simulink model "Visualization"  (R2015a)
settings: Solver=FixedStepDiscrete  SolverMode=SingleTasking  StartTime=0.0  StopTime=inf  FixedStep=0.001  MaxStep=0.004  RelTol=1e-3
undefined symbols (not defined in the file or in its folder): gcbh, vrmfunc
libraries: dspsigops x2
settings Model: CovSFcnEnable=off  Creator=ADAM  LastModifiedBy=denise
settings SolverCC: ExtrapolationOrder=1
settings DataIOCC: LimitDataPoints=off  MaxDataPoints=1  SaveFormat=Structure  SignalLoggingSaveFormat=ModelDataLogs  SaveOutput=off  SignalLogging=off  DSMLogging=off  SaveTime=off  OutputSaveName=model_out  SignalLoggingName=model_out
settings OptimizationCC: ExpressionDepthLimit=2147483647  SimCompilerOptimization=on
settings DebuggingCC: UnderspecifiedInitializationDetection=Classic  MergeDetectMultiDrivingBlocksExec=none  SolverPrmCheckMsg=warning  InheritedTsInSrcMsg=none  MultiTaskDSMMsg=warning  MultiTaskCondExecSysMsg=none  UnconnectedInputMsg=none  UnconnectedOutputMsg=none  UnconnectedLineMsg=none  StateNameClashWarn=warning
settings HardwareCC: ProdIntDivRoundTo=Zero  ProdEndianess=LittleEndian  ProdHWDeviceType=Generic->32-bit x86 compatible
settings CodeAppCC: MaxIdLength=95

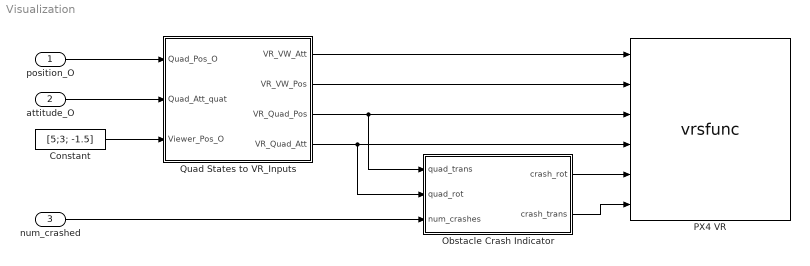
== system Visualization ==
  position_O : Inport  OutDataTypeStr=double  PortDimensions=3  SampleTime=0
  attitude_O : Inport  Port=2  OutDataTypeStr=double  PortDimensions=4  SampleTime=0
  num_crashed : Inport  Port=3  OutDataTypeStr=double  PortDimensions=1  SampleTime=0
  Constant : Constant  Value=[5;3; -1.5]  VectorParams1D=off
  Obstacle Crash Indicator : Subsystem
  PX4 VR : S-Function  InstantiateOnLoad=on  LoadFcn=vrmfunc('FnLoad', gcbh);  InitFcn=vrmfunc('FnInit', gcbh);  StartFcn=vrmfunc('FnSimStatus', gcbh, 'running')  StopFcn=vrmfunc('FnStop', gcbh)  FunctionName=vrsfunc  Parameters=SampleTime, VideoDimensions, 0  mask(Virtual Reality Sink){SampleTime=0.04, ViewEnable=on, RemoteChange=off, RemoteView=off, FieldsWritten=VW_Standing.orientation.4.1.1.double#VW_Standing.position.3.1.1.double#Quad_group.translation.3.1.1.double#Quad.rotation.4.1.1.double#crash.rotation.4.1.1.double#crash.translation.3.1.1.double, WorldFileName=px4.wrl, WorldDescription=TUW Field, AutoView=off, VideoDimensions=[], AllowVariableSize=off, FigureProperties=}
      mask prompts: SampleTime "Sample Time"; ViewEnable "View"; RemoteChange "Remote Change"; RemoteView "Remote View"; FieldsWritten "Fields Written"; WorldFileName "World File Name"; WorldDescription "World Description"; VideoDimensions "Video Dimensions"; AllowVariableSize "Allow Variable Size"; FigureProperties "Figure Properties"
      mask help: Controls the selected fields of a virtual world according to given inputs.
      mask init:
      | set_param(gcbh, 'MaskDisplay', vrmfunc('FnIcon'));
      settings: CopyFcn=vrmfunc('FnCopy', gcbh);  DeleteFcn=vrmfunc('FnDelete', gcbh);  PreSaveFcn=vrmfunc('FnPreSave', gcbh);  PauseFcn=vrmfunc('FnSimStatus', gcbh, 'paused');  ContinueFcn=vrmfunc('FnSimStatus', gcbh, 'running');  DestroyFcn=vrmfunc('FnDestroy', gcbh);  OpenFcn=vrmfunc('FnOpen', gcbh);  CloseFcn=vrmfunc('FnClose', gcbh);
      mask Help: helpview(vrmfunc('FnHelpTopic'), 'vr_vrsink');
      mask Display:
      | image(imread('vrblockicon.png'));
      | port_label('input', 1, 'VW_Standing.orientation');
      | port_label('input', 2, 'VW_Standing.position');
      | port_label('input', 3, 'Quad_group.translation');
      | port_label('input', 4, 'Quad.rotation');
      | port_label('input', 5, 'crash.rotation');
      | port_label('input', 6, 'crash.translation');
  Quad States to VR_Inputs : Subsystem
  wires:
  Constant/1 -> Quad States to VR_Inputs/3(Viewer_Pos_O)
  position_O/1 -> Quad States to VR_Inputs/1(Quad_Pos_O)
  attitude_O/1 -> Quad States to VR_Inputs/2(Quad_Att_quat)
  Quad States to VR_Inputs/1(VR_VW_Att) -> PX4 VR/1
  Quad States to VR_Inputs/2(VR_VW_Pos) -> PX4 VR/2
  Quad States to VR_Inputs/3(VR_Quad_Pos) -> Obstacle Crash Indicator/1(quad_trans), PX4 VR/3
  Quad States to VR_Inputs/4(VR_Quad_Att) -> Obstacle Crash Indicator/2(quad_rot), PX4 VR/4
  num_crashed/1 -> Obstacle Crash Indicator/3(num_crashes)
  Obstacle Crash Indicator/2(crash_trans) -> PX4 VR/6
  Obstacle Crash Indicator/1(crash_rot) -> PX4 VR/5

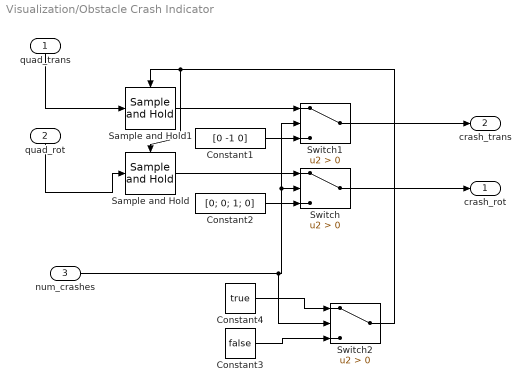
== system Visualization/Obstacle Crash Indicator ==
  quad_trans : Inport
  quad_rot : Inport  Port=2
  num_crashes : Inport  Port=3
  Constant1 : Constant  Value=[0 -1 0]  VectorParams1D=off
  Constant2 : Constant  Value=[0; 0; 1; 0]  VectorParams1D=off
  Constant3 : Constant  Value=false
  Constant4 : Constant  Value=true
  Sample and Hold : dspsigops/Sample and Hold  trig=Rising edge  initCond=0  latchinput=off
  Sample and Hold1 : dspsigops/Sample and Hold  trig=Rising edge  initCond=0  latchinput=off
  Switch : Switch  Criteria=u2 > Threshold
  Switch1 : Switch  Criteria=u2 > Threshold
  Switch2 : Switch  Criteria=u2 > Threshold
  crash_rot : Outport
  crash_trans : Outport  Port=2
  wires:
  Sample and Hold/1 -> Switch/1
  quad_trans/1 -> Sample and Hold1/1
  Constant4/1 -> Switch2/1
  Sample and Hold1/1 -> Switch1/1
  Constant3/1 -> Switch2/3
  Constant1/1 -> Switch1/3
  Switch1/1 -> crash_trans/1
  num_crashes/1 -> Switch2/2, Switch1/2, Switch/2
  Constant2/1 -> Switch/3
  Switch/1 -> crash_rot/1
  Switch2/1 -> Sample and Hold1/Trigger, Sample and Hold/Trigger
  quad_rot/1 -> Sample and Hold/1

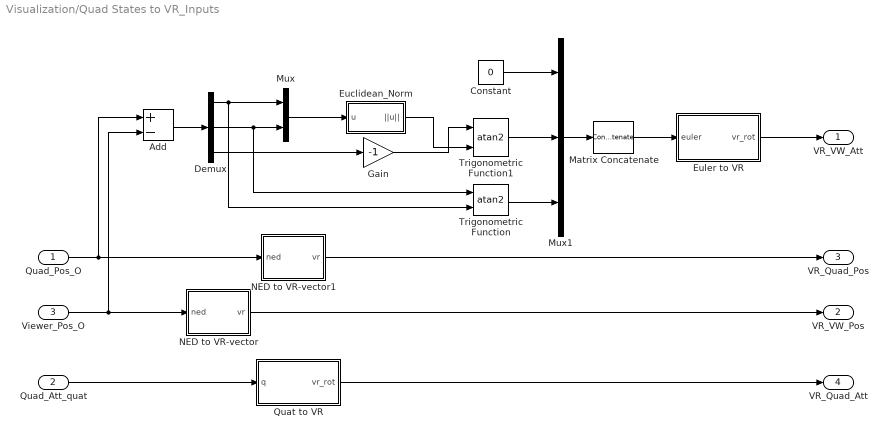
== system Visualization/Quad States to VR_Inputs ==
  Quad_Pos_O : Inport
  Quad_Att_quat : Inport  Port=2
  Viewer_Pos_O : Inport  Port=3
  Add : Sum  Inputs=+-
  Constant : Constant  Value=0
  Demux : Demux  Outputs=3
  Euclidean_Norm : Subsystem
      mask help: Euclidean Norm
      mask Help: Euclidean Norm
      mask Display: disp('||.||')
  Euler to VR : Subsystem  mask(Euler oritentation to VR-rotation){}
      mask help:
      | Converts a vector of euler angles to a VR-rotation.
      |
      | 1st rotation: psi   (=eul(1)) around z
      | 2nd rotation: theta (=eul(2)) around y
      | 3rd rotation: phi   (=eul(3)) around x
  Gain : Gain  Gain=-1
  Matrix Concatenate : Concatenate  NumInputs=1  Mode=Multidimensional array
  Mux : Mux  Inputs=2
  Mux1 : Mux  Inputs=3
  NED to VR-vector : Subsystem  mask(Converts NED to VR-vector){}
      mask help: [north east down] => [east up south]
  NED to VR-vector1 : Subsystem  mask(Converts NED to VR-vector){}
      mask help: [north east down] => [east up south]
  Quat to VR : Subsystem  mask(Quaternion to VR-rotation){}
      mask help: Converts a normalized quaternion to a VR-rotation.
  Trigonometric Function : Trigonometry  Operator=atan2
  Trigonometric Function1 : Trigonometry  Operator=atan2
  VR_VW_Att : Outport
  VR_VW_Pos : Outport  Port=2
  VR_Quad_Pos : Outport  Port=3
  VR_Quad_Att : Outport  Port=4
  wires:
  Trigonometric Function1/1 -> Mux1/2
  Trigonometric Function/1 -> Mux1/3
  Constant/1 -> Mux1/1
  Matrix Concatenate/1 -> Euler to VR/1(euler)
  Gain/1 -> Trigonometric Function1/1
  Demux/3 -> Gain/1
  Demux/1 -> Mux/1, Trigonometric Function/2
  Demux/2 -> Mux/2, Trigonometric Function/1
  NED to VR-vector/1(vr) -> VR_VW_Pos/1
  NED to VR-vector1/1(vr) -> VR_Quad_Pos/1
  Mux1/1 -> Matrix Concatenate/1
  Euler to VR/1(vr_rot) -> VR_VW_Att/1
  Mux/1 -> Euclidean_Norm/1(u)
  Euclidean_Norm/1(||u||) -> Trigonometric Function1/2
  Add/1 -> Demux/1
  Quad_Pos_O/1 -> Add/1, NED to VR-vector1/1(ned)
  Quat to VR/1(vr_rot) -> VR_Quad_Att/1
  Quad_Att_quat/1 -> Quat to VR/1(q)
  Viewer_Pos_O/1 -> Add/2, NED to VR-vector/1(ned)

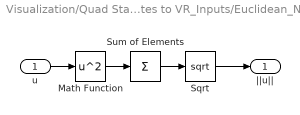
== system Visualization/Quad States to VR_Inputs/Euclidean_Norm ==
  u : Inport
  Math Function : Math  Operator=square  SaturateOnIntegerOverflow=on
  Sqrt : Sqrt  SaturateOnIntegerOverflow=on
  Sum of Elements : Sum  Inputs=+
  ||u|| : Outport
  wires:
  Sqrt/1 -> ||u||/1
  Sum of Elements/1 -> Sqrt/1
  Math Function/1 -> Sum of Elements/1
  u/1 -> Math Function/1

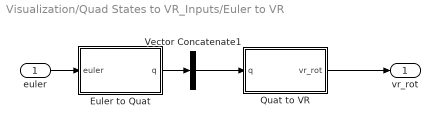
== system Visualization/Quad States to VR_Inputs/Euler to VR ==
  euler : Inport
  Euler to Quat : Subsystem  mask(Euler angles to Quaternion){}
      mask help:
      | vector [phi; theta; psi] means:
      | 1. rotation: psi   (=eul(3)) around z axis
      | 2. rotation: theta (=eul(2)) around y axis
      | 3. rotation: phi   (=eul(1)) around x axis
      |
      | Regrettably implemented in Simulink
  Quat to VR : Subsystem  mask(Quaternion to VR-rotation){}
      mask help: Converts a normalized quaternion to a VR-rotation.
  Vector Concatenate1 : Concatenate  NumInputs=1  Mode=Multidimensional array
  vr_rot : Outport
  wires:
  Quat to VR/1(vr_rot) -> vr_rot/1
  Euler to Quat/1(q) -> Vector Concatenate1/1
  euler/1 -> Euler to Quat/1(euler)
  Vector Concatenate1/1 -> Quat to VR/1(q)

== system Visualization/Quad States to VR_Inputs/NED to VR-vector ==
  ned : Inport
  Gain K*u : Gain  Gain=[0 1 0; 0 0 -1; -1 0 0]  Multiplication=Matrix(K*u)
  vr : Outport
  wires:
  Gain K*u/1 -> vr/1
  ned/1 -> Gain K*u/1

== system Visualization/Quad States to VR_Inputs/NED to VR-vector1 ==
  ned : Inport
  Gain K*u : Gain  Gain=[0 1 0; 0 0 -1; -1 0 0]  Multiplication=Matrix(K*u)
  vr : Outport
  wires:
  Gain K*u/1 -> vr/1
  ned/1 -> Gain K*u/1

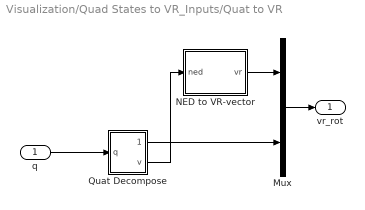
== system Visualization/Quad States to VR_Inputs/Quat to VR ==
  q : Inport
  Mux : Mux  Inputs=2
  NED to VR-vector : Subsystem  mask(Converts NED to VR-vector){}
      mask help: [north east down] => [east up south]
  Quat Decompose : Subsystem  mask(Quaternion Decomposition){}
      mask help:
      | Decomposes a normalized Quaternion into
      | the rotation-vector v and the rotation-angle phi.
  vr_rot : Outport
  wires:
  q/1 -> Quat Decompose/1(q)
  Quat Decompose/2(v) -> NED to VR-vector/1(ned)
  NED to VR-vector/1(vr) -> Mux/1
  Quat Decompose/1(phi) -> Mux/2
  Mux/1 -> vr_rot/1

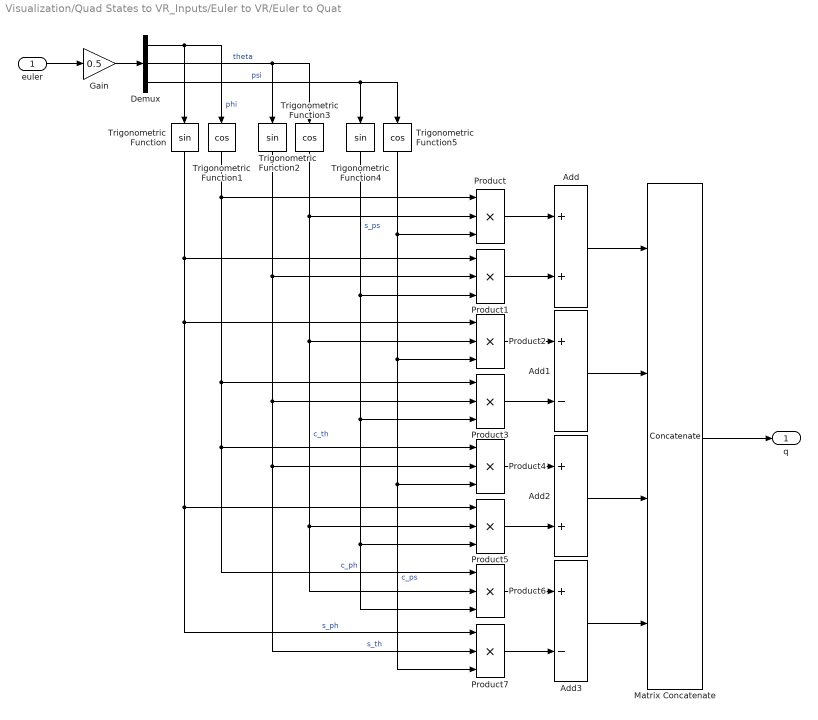
== system Visualization/Quad States to VR_Inputs/Euler to VR/Euler to Quat ==
  euler : Inport
  Add : Sum
  Add1 : Sum  Inputs=+-
  Add2 : Sum
  Add3 : Sum  Inputs=+-
  Demux : Demux  Outputs=3
  Gain : Gain  Gain=0.5
  Matrix Concatenate : Concatenate  NumInputs=4  ConcatenateDimension=2
  Product{,1..7} (8 alike) : Product  Inputs=3  RndMeth=Zero
  Trigonometric Function : Trigonometry
  Trigonometric Function1 : Trigonometry  Operator=cos
  Trigonometric Function2 : Trigonometry
  Trigonometric Function3 : Trigonometry  Operator=cos
  Trigonometric Function4 : Trigonometry
  Trigonometric Function5 : Trigonometry  Operator=cos
  q : Outport
  wires:
  Trigonometric Function1/1 -> Product/1, Product3/1, Product4/1, Product6/1  "c_ph"
  Trigonometric Function3/1 -> Product/2, Product2/2, Product5/2, Product6/2  "c_th"
  Trigonometric Function4/1 -> Product1/3, Product3/3, Product5/3, Product6/3  "s_ps"
  Trigonometric Function/1 -> Product1/1, Product2/1, Product5/1, Product7/1  "s_ph"
  Trigonometric Function2/1 -> Product1/2, Product3/2, Product4/2, Product7/2  "s_th"
  Trigonometric Function5/1 -> Product/3, Product2/3, Product4/3, Product7/3  "c_ps"
  Matrix Concatenate/1 -> q/1
  Add3/1 -> Matrix Concatenate/4
  Add2/1 -> Matrix Concatenate/3
  Add1/1 -> Matrix Concatenate/2
  Add/1 -> Matrix Concatenate/1
  Product7/1 -> Add3/2
  Product6/1 -> Add3/1
  Product5/1 -> Add2/2
  Product4/1 -> Add2/1
  Product3/1 -> Add1/2
  Product2/1 -> Add1/1
  Product1/1 -> Add/2
  Product/1 -> Add/1
  Demux/1 -> Trigonometric Function1/1, Trigonometric Function/1  "phi"
  Demux/2 -> Trigonometric Function3/1, Trigonometric Function2/1  "theta"
  Demux/3 -> Trigonometric Function5/1, Trigonometric Function4/1  "psi"
  Gain/1 -> Demux/1
  euler/1 -> Gain/1

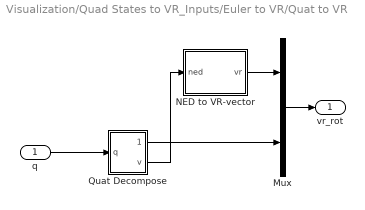
== system Visualization/Quad States to VR_Inputs/Euler to VR/Quat to VR ==
  q : Inport
  Mux : Mux  Inputs=2
  NED to VR-vector : Subsystem  mask(Converts NED to VR-vector){}
      mask help: [north east down] => [east up south]
  Quat Decompose : Subsystem  mask(Quaternion Decomposition){}
      mask help:
      | Decomposes a normalized Quaternion into
      | the rotation-vector v and the rotation-angle phi.
  vr_rot : Outport
  wires:
  q/1 -> Quat Decompose/1(q)
  Quat Decompose/2(v) -> NED to VR-vector/1(ned)
  NED to VR-vector/1(vr) -> Mux/1
  Quat Decompose/1(phi) -> Mux/2
  Mux/1 -> vr_rot/1

== system Visualization/Quad States to VR_Inputs/Quat to VR/NED to VR-vector ==
  ned : Inport
  Gain K*u : Gain  Gain=[0 1 0; 0 0 -1; -1 0 0]  Multiplication=Matrix(K*u)
  vr : Outport
  wires:
  Gain K*u/1 -> vr/1
  ned/1 -> Gain K*u/1

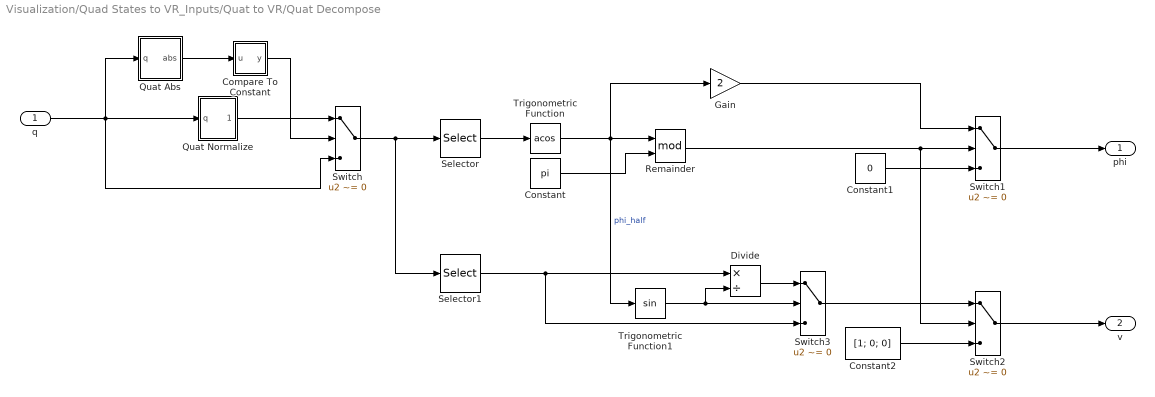
== system Visualization/Quad States to VR_Inputs/Quat to VR/Quat Decompose ==
  q : Inport
  Compare To Constant : Subsystem  mask(Compare To Constant){relop=~=, const=1, OutDataTypeStr=uint8, ZeroCross=off}
      mask prompts: relop "Simulink:masks:Operator_MP"; const "Simulink:masks:ConstantValue_MP"; OutDataTypeStr "Simulink:masks:OutputDataType_MP"; ZeroCross "Simulink:masks:EnableZerocrossingDetection_MP"
      mask help: Simulink:masks:CompareToConstant_MD
      mask init:
      | blkName = gcb;
      | 
      | if strcmp(get_param(gcbh,'OutDataTypeStr'),'boolean')
      | 	setValue = 'boolean';
      | else
      | 	setValue = 'fixdt(0, 8)';
      | end
      | 
      | set_param([blkName,'/Compare'],'relop',relop, ...
      | 	'OutDataTypeStr', setValue, 'ZeroCross', ZeroCross);
      | 
      | str = [relop,' C']; %default
      | 
      | const_str = get_param(blkName, 'const');
      | 
      | if isempty(strfind(const_str, ' ')) && isempty(strfind(const_str, ','))
      |     % scalar or single expression
      |     if isempty(str2num(const_str))
      |         %expression
      |         str = [relop, ' ', const_str];
      |     elseif length(const) == 1
      |         str = [relop,' ',num2str(double(const))];
      |     end
      | end
      mask TypeOptions relop: == | ~= | < | <= | >= | >
      mask TypeOptions OutDataTypeStr: Simulink:masks:uint8 | Simulink:masks:boolean
      mask Callback ZeroCross: sl('zeroCrossEnable', gcbh);
      mask Display: disp(str)
  Constant : Constant  Value=pi  OutDataTypeStr=Inherit: Inherit via back propagation
  Constant1 : Constant  Value=0  VectorParams1D=off
  Constant2 : Constant  Value=[1; 0; 0]  VectorParams1D=off
  Divide : Product  Inputs=*/
  Gain : Gain  Gain=2
  Quat Abs : Subsystem  mask(Absolute value){}
      mask help: sqrt(q(1)^2+q(2)^2+q(3)^2+q(4)^2)
      mask init:
      | pos = get_param(gcb, 'Position');
      | width = pos(3) - pos(1); height = pos(4) - pos(2);
      | fontsize = get_param(gcb, 'fontsize');
      | if fontsize==-1, scale=1; else scale=fontsize/10; end
      mask Display: text(width/2-scale*8, (height/2-scale), '||q||')
  Quat Normalize : Subsystem  mask(Quaternion Normalize){}
      mask help:
      | if abs(q) ~= 0
      |     q_norm = q/sqrt(q(1)^2+q(2)^2+q(3)^2+q(4)^2)
      | else
      |     q_norm = [1; 0; 0; 0]
      |
      | Regrettably implemented in Simulink
      mask init:
      | pos = get_param(gcb, 'Position');
      | width = pos(3) - pos(1); height = pos(4) - pos(2);
      | fontsize = get_param(gcb, 'fontsize');
      | if fontsize==-1, scale=1; else scale=fontsize/10; end
      mask Display:
      | text(width/2-scale*3, (height/2+scale*10), 'q')
      | text(width/2-scale*8, (height/2-scale*6), '||q||')
      | plot([width/2-scale*10 width/2+scale*10], height/2*[1 1])
  Remainder : Math  Operator=mod  SaturateOnIntegerOverflow=on
  Selector : Selector  InputPortWidth=4  Indices=[1]
  Selector1 : Selector  InputPortWidth=4  Indices=[2 3 4]
  Switch{,1..3} (4 alike) : Switch  Criteria=u2 ~= 0
  Trigonometric Function : Trigonometry  Operator=acos
  Trigonometric Function1 : Trigonometry
  phi : Outport
  v : Outport  Port=2
  wires:
  q/1 -> Switch/3, Quat Abs/1(q), Quat Normalize/1(q)
  Quat Abs/1(abs) -> Compare To Constant/1(u)
  Compare To Constant/1(y) -> Switch/2
  Quat Normalize/1(q_norm) -> Switch/1
  Switch/1 -> Selector/1, Selector1/1
  Selector/1 -> Trigonometric Function/1
  Trigonometric Function/1 -> Remainder/1, Gain/1, Trigonometric Function1/1  "phi_half"
  Constant/1 -> Remainder/2
  Remainder/1 -> Switch1/2, Switch2/2
  Gain/1 -> Switch1/1
  Switch1/1 -> phi/1
  Switch2/1 -> v/1
  Constant1/1 -> Switch1/3
  Constant2/1 -> Switch2/3
  Trigonometric Function1/1 -> Switch3/2, Divide/2
  Switch3/1 -> Switch2/1
  Selector1/1 -> Divide/1, Switch3/3
  Divide/1 -> Switch3/1

== system Visualization/Quad States to VR_Inputs/Euler to VR/Quat to VR/NED to VR-vector ==
  ned : Inport
  Gain K*u : Gain  Gain=[0 1 0; 0 0 -1; -1 0 0]  Multiplication=Matrix(K*u)
  vr : Outport
  wires:
  Gain K*u/1 -> vr/1
  ned/1 -> Gain K*u/1

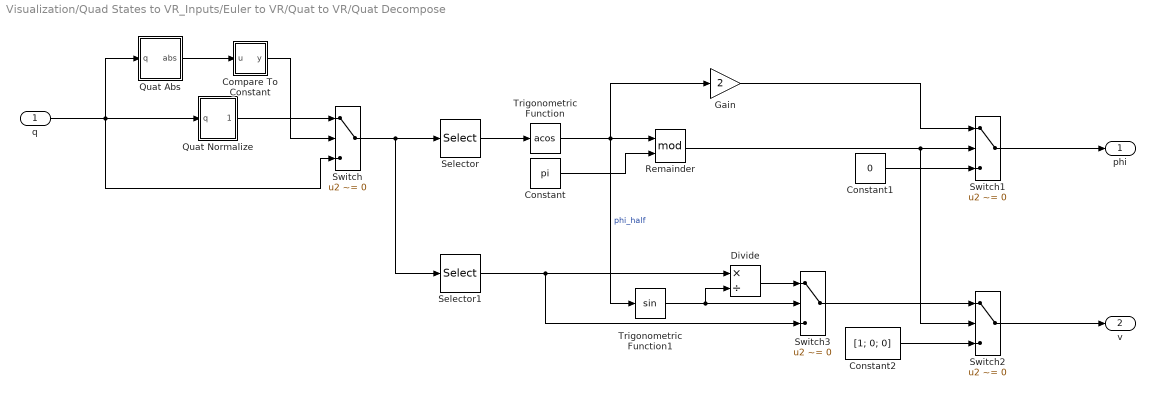
== system Visualization/Quad States to VR_Inputs/Euler to VR/Quat to VR/Quat Decompose ==
  q : Inport
  Compare To Constant : Subsystem  mask(Compare To Constant){relop=~=, const=1, OutDataTypeStr=uint8, ZeroCross=off}
      mask prompts: relop "Simulink:masks:Operator_MP"; const "Simulink:masks:ConstantValue_MP"; OutDataTypeStr "Simulink:masks:OutputDataType_MP"; ZeroCross "Simulink:masks:EnableZerocrossingDetection_MP"
      mask help: Simulink:masks:CompareToConstant_MD
      mask init: same as Visualization/Quad States to VR_Inputs/Quat to VR/Quat Decompose/Compare To Constant
      mask TypeOptions relop: == | ~= | < | <= | >= | >
      mask TypeOptions OutDataTypeStr: Simulink:masks:uint8 | Simulink:masks:boolean
      mask Callback ZeroCross: sl('zeroCrossEnable', gcbh);
      mask Display: disp(str)
  Constant : Constant  Value=pi  OutDataTypeStr=Inherit: Inherit via back propagation
  Constant1 : Constant  Value=0  VectorParams1D=off
  Constant2 : Constant  Value=[1; 0; 0]  VectorParams1D=off
  Divide : Product  Inputs=*/
  Gain : Gain  Gain=2
  Quat Abs : Subsystem  mask(Absolute value){}
      mask help: sqrt(q(1)^2+q(2)^2+q(3)^2+q(4)^2)
      mask init:
      | pos = get_param(gcb, 'Position');
      | width = pos(3) - pos(1); height = pos(4) - pos(2);
      | fontsize = get_param(gcb, 'fontsize');
      | if fontsize==-1, scale=1; else scale=fontsize/10; end
      mask Display: text(width/2-scale*8, (height/2-scale), '||q||')
  Quat Normalize : Subsystem  mask(Quaternion Normalize){}
      mask help:
      | if abs(q) ~= 0
      |     q_norm = q/sqrt(q(1)^2+q(2)^2+q(3)^2+q(4)^2)
      | else
      |     q_norm = [1; 0; 0; 0]
      |
      | Regrettably implemented in Simulink
      mask init:
      | pos = get_param(gcb, 'Position');
      | width = pos(3) - pos(1); height = pos(4) - pos(2);
      | fontsize = get_param(gcb, 'fontsize');
      | if fontsize==-1, scale=1; else scale=fontsize/10; end
      mask Display:
      | text(width/2-scale*3, (height/2+scale*10), 'q')
      | text(width/2-scale*8, (height/2-scale*6), '||q||')
      | plot([width/2-scale*10 width/2+scale*10], height/2*[1 1])
  Remainder : Math  Operator=mod  SaturateOnIntegerOverflow=on
  Selector : Selector  InputPortWidth=4  Indices=[1]
  Selector1 : Selector  InputPortWidth=4  Indices=[2 3 4]
  Switch{,1..3} (4 alike) : Switch  Criteria=u2 ~= 0
  Trigonometric Function : Trigonometry  Operator=acos
  Trigonometric Function1 : Trigonometry
  phi : Outport
  v : Outport  Port=2
  wires:
  q/1 -> Switch/3, Quat Abs/1(q), Quat Normalize/1(q)
  Quat Abs/1(abs) -> Compare To Constant/1(u)
  Compare To Constant/1(y) -> Switch/2
  Quat Normalize/1(q_norm) -> Switch/1
  Switch/1 -> Selector/1, Selector1/1
  Selector/1 -> Trigonometric Function/1
  Trigonometric Function/1 -> Remainder/1, Gain/1, Trigonometric Function1/1  "phi_half"
  Constant/1 -> Remainder/2
  Remainder/1 -> Switch1/2, Switch2/2
  Gain/1 -> Switch1/1
  Switch1/1 -> phi/1
  Switch2/1 -> v/1
  Constant1/1 -> Switch1/3
  Constant2/1 -> Switch2/3
  Trigonometric Function1/1 -> Switch3/2, Divide/2
  Switch3/1 -> Switch2/1
  Selector1/1 -> Divide/1, Switch3/3
  Divide/1 -> Switch3/1

== system Visualization/Quad States to VR_Inputs/Quat to VR/Quat Decompose/Compare To Constant ==
  u : Inport
  Compare : RelationalOperator  Operator=~=  OutDataTypeStr=fixdt(0, 8)  ZeroCross=off  InputSameDT=on
  Constant : Constant  DisableCoverage=on  Value=const  OutDataTypeStr=Inherit: Inherit via back propagation
  y : Outport
  wires:
  Compare/1 -> y/1
  Constant/1 -> Compare/2
  u/1 -> Compare/1

== system Visualization/Quad States to VR_Inputs/Quat to VR/Quat Decompose/Quat Abs ==
  q : Inport
  Euclidean_Norm : Subsystem
      mask help: Euclidean Norm
      mask Help: Euclidean Norm
      mask Display: disp('||.||')
  abs : Outport
  wires:
  q/1 -> Euclidean_Norm/1(u)
  Euclidean_Norm/1(||u||) -> abs/1

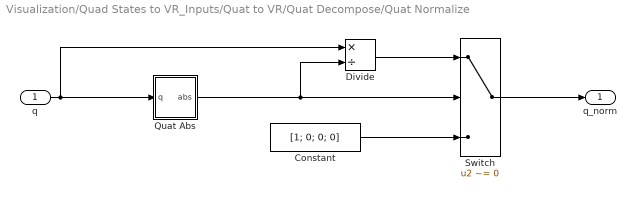
== system Visualization/Quad States to VR_Inputs/Quat to VR/Quat Decompose/Quat Normalize ==
  q : Inport
  Constant : Constant  Value=[1; 0; 0; 0]  VectorParams1D=off  OutDataTypeStr=Inherit: Inherit via back propagation
  Divide : Product  Inputs=*/  OutMin=-1.5  OutMax=1.5  OutDataTypeStr=Inherit: Same as first input
  Quat Abs : Subsystem  mask(Absolute value){}
      mask help: sqrt(q(1)^2+q(2)^2+q(3)^2+q(4)^2)
      mask init:
      | pos = get_param(gcb, 'Position');
      | width = pos(3) - pos(1); height = pos(4) - pos(2);
      | fontsize = get_param(gcb, 'fontsize');
      | if fontsize==-1, scale=1; else scale=fontsize/10; end
      mask Display: text(width/2-scale*8, (height/2-scale), '||q||')
  Switch : Switch  Criteria=u2 ~= 0
  q_norm : Outport
  wires:
  Constant/1 -> Switch/3
  Divide/1 -> Switch/1
  Quat Abs/1(abs) -> Divide/2, Switch/2
  q/1 -> Divide/1, Quat Abs/1(q)
  Switch/1 -> q_norm/1

== system Visualization/Quad States to VR_Inputs/Euler to VR/Quat to VR/Quat Decompose/Compare To Constant ==
  u : Inport
  Compare : RelationalOperator  Operator=~=  OutDataTypeStr=fixdt(0, 8)  ZeroCross=off  InputSameDT=on
  Constant : Constant  DisableCoverage=on  Value=const  OutDataTypeStr=Inherit: Inherit via back propagation
  y : Outport
  wires:
  Compare/1 -> y/1
  Constant/1 -> Compare/2
  u/1 -> Compare/1

== system Visualization/Quad States to VR_Inputs/Euler to VR/Quat to VR/Quat Decompose/Quat Abs ==
  q : Inport
  Euclidean_Norm : Subsystem
      mask help: Euclidean Norm
      mask Help: Euclidean Norm
      mask Display: disp('||.||')
  abs : Outport
  wires:
  q/1 -> Euclidean_Norm/1(u)
  Euclidean_Norm/1(||u||) -> abs/1

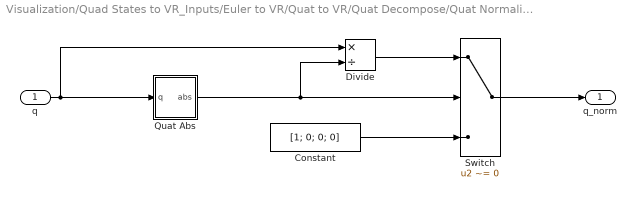
== system Visualization/Quad States to VR_Inputs/Euler to VR/Quat to VR/Quat Decompose/Quat Normalize ==
  q : Inport
  Constant : Constant  Value=[1; 0; 0; 0]  VectorParams1D=off  OutDataTypeStr=Inherit: Inherit via back propagation
  Divide : Product  Inputs=*/  OutMin=-1.5  OutMax=1.5  OutDataTypeStr=Inherit: Same as first input
  Quat Abs : Subsystem  mask(Absolute value){}
      mask help: sqrt(q(1)^2+q(2)^2+q(3)^2+q(4)^2)
      mask init:
      | pos = get_param(gcb, 'Position');
      | width = pos(3) - pos(1); height = pos(4) - pos(2);
      | fontsize = get_param(gcb, 'fontsize');
      | if fontsize==-1, scale=1; else scale=fontsize/10; end
      mask Display: text(width/2-scale*8, (height/2-scale), '||q||')
  Switch : Switch  Criteria=u2 ~= 0
  q_norm : Outport
  wires:
  Constant/1 -> Switch/3
  Divide/1 -> Switch/1
  Quat Abs/1(abs) -> Divide/2, Switch/2
  q/1 -> Divide/1, Quat Abs/1(q)
  Switch/1 -> q_norm/1

== system Visualization/Quad States to VR_Inputs/Quat to VR/Quat Decompose/Quat Abs/Euclidean_Norm ==
  u : Inport
  Math Function : Math  Operator=square  SaturateOnIntegerOverflow=on
  Sqrt : Sqrt  SaturateOnIntegerOverflow=on
  Sum of Elements : Sum  Inputs=+
  ||u|| : Outport
  wires:
  Sqrt/1 -> ||u||/1
  Sum of Elements/1 -> Sqrt/1
  Math Function/1 -> Sum of Elements/1
  u/1 -> Math Function/1

== system Visualization/Quad States to VR_Inputs/Quat to VR/Quat Decompose/Quat Normalize/Quat Abs ==
  q : Inport
  Euclidean_Norm : Subsystem
      mask help: Euclidean Norm
      mask Help: Euclidean Norm
      mask Display: disp('||.||')
  abs : Outport
  wires:
  q/1 -> Euclidean_Norm/1(u)
  Euclidean_Norm/1(||u||) -> abs/1

== system Visualization/Quad States to VR_Inputs/Euler to VR/Quat to VR/Quat Decompose/Quat Abs/Euclidean_Norm ==
  u : Inport
  Math Function : Math  Operator=square  SaturateOnIntegerOverflow=on
  Sqrt : Sqrt  SaturateOnIntegerOverflow=on
  Sum of Elements : Sum  Inputs=+
  ||u|| : Outport
  wires:
  Sqrt/1 -> ||u||/1
  Sum of Elements/1 -> Sqrt/1
  Math Function/1 -> Sum of Elements/1
  u/1 -> Math Function/1

== system Visualization/Quad States to VR_Inputs/Euler to VR/Quat to VR/Quat Decompose/Quat Normalize/Quat Abs ==
  q : Inport
  Euclidean_Norm : Subsystem
      mask help: Euclidean Norm
      mask Help: Euclidean Norm
      mask Display: disp('||.||')
  abs : Outport
  wires:
  q/1 -> Euclidean_Norm/1(u)
  Euclidean_Norm/1(||u||) -> abs/1

== system Visualization/Quad States to VR_Inputs/Quat to VR/Quat Decompose/Quat Normalize/Quat Abs/Euclidean_Norm ==
  u : Inport
  Math Function : Math  Operator=square  SaturateOnIntegerOverflow=on
  Sqrt : Sqrt  SaturateOnIntegerOverflow=on
  Sum of Elements : Sum  Inputs=+
  ||u|| : Outport
  wires:
  Sqrt/1 -> ||u||/1
  Sum of Elements/1 -> Sqrt/1
  Math Function/1 -> Sum of Elements/1
  u/1 -> Math Function/1

== system Visualization/Quad States to VR_Inputs/Euler to VR/Quat to VR/Quat Decompose/Quat Normalize/Quat Abs/Euclidean_Norm ==
  u : Inport
  Math Function : Math  Operator=square  SaturateOnIntegerOverflow=on
  Sqrt : Sqrt  SaturateOnIntegerOverflow=on
  Sum of Elements : Sum  Inputs=+
  ||u|| : Outport
  wires:
  Sqrt/1 -> ||u||/1
  Sum of Elements/1 -> Sqrt/1
  Math Function/1 -> Sum of Elements/1
  u/1 -> Math Function/1
